simulink model "qdr_ct_test"  (R2012b)
settings: Solver=ode45  StartTime=0.0  StopTime=50000  RelTol=1e-3
libraries: xbsIndex_r4 x1070, casper_library_misc x5, xps_library x4, casper_library_delays x4
(part 1 of 10)
settings Model: Creator=jackh  LastModifiedBy=jackh

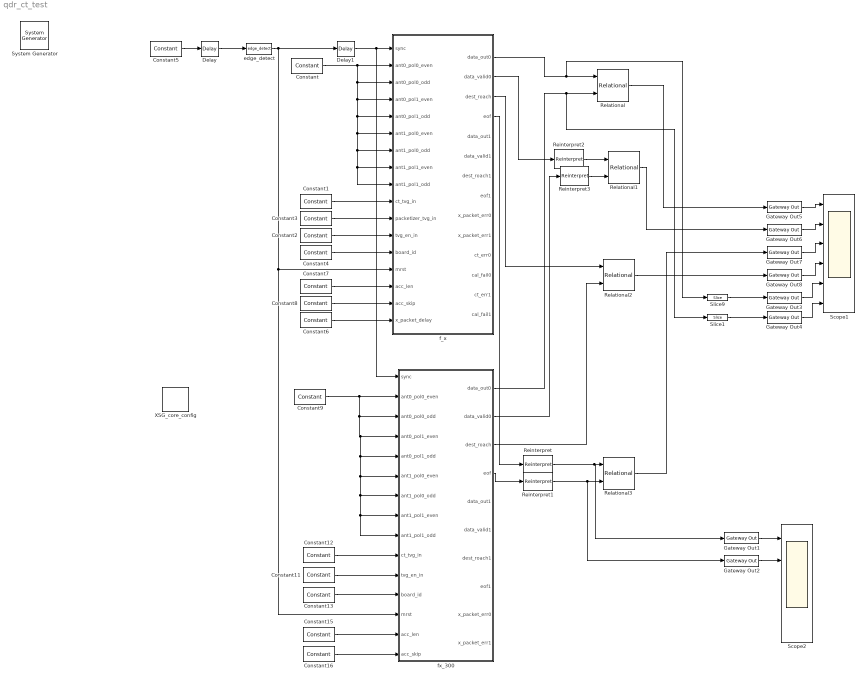
== system qdr_ct_test ==
  " System Generator" : xbsIndex_r4/ System Generator  Tag=genX  xilinxfamily=Kintex7  part=xc7k325t  speed=-3  package=fbg676  synthesis_tool=XST  clock_wrapper=Clock Enables  directory=./netlist  proj_type=Project Navigator  Synth_file=XST Defaults  Impl_file=ISE Defaults  testbench=off  simulink_period=1  sysclk_period=10  dcm_input_clock_period=10  incr_netlist=off  trim_vbits=Everywhere in SubSystem  dbl_ovrd=According to Block Masks  core_generation=According to Block Masks  run_coregen=off  deprecated_control=off  eval_field=0  block_type=sysgen
  Constant{,4,6,9,13} (5 alike) : xbsIndex_r4/Constant  const=0  gui_display_data_type=Fixed-point  arith_type=Unsigned  n_bits=8  bin_pt=0  preci_type=Single  exp_width=8  frac_width=24  explicit_period=on  period=1  equ=P=C  opselect=C  inp2=PCIN>>17  opr=+  inp1=P  carry=CIN  dbl_ovrd=off  block_type=constant
  Constant{1..3,5,11..12} (6 alike) : xbsIndex_r4/Constant  const=1  gui_display_data_type=Boolean  arith_type=Boolean  n_bits=8  bin_pt=0  preci_type=Single  exp_width=8  frac_width=24  explicit_period=on  period=1  equ=P=C  opselect=C  inp2=PCIN>>17  opr=+  inp1=P  carry=CIN  dbl_ovrd=off  block_type=constant
  Constant15 : xbsIndex_r4/Constant  const=64  gui_display_data_type=Fixed-point  arith_type=Unsigned  n_bits=16  bin_pt=0  preci_type=Single  exp_width=8  frac_width=24  explicit_period=on  period=1  equ=P=C  opselect=C  inp2=PCIN>>17  opr=+  inp1=P  carry=CIN  dbl_ovrd=off  block_type=constant
  Constant16 : xbsIndex_r4/Constant  const=10  gui_display_data_type=Fixed-point  arith_type=Unsigned  n_bits=16  bin_pt=0  preci_type=Single  exp_width=8  frac_width=24  explicit_period=on  period=1  equ=P=C  opselect=C  inp2=PCIN>>17  opr=+  inp1=P  carry=CIN  dbl_ovrd=off  block_type=constant
  Constant7 : xbsIndex_r4/Constant  const=32*2  gui_display_data_type=Fixed-point  arith_type=Unsigned  n_bits=16  bin_pt=0  preci_type=Single  exp_width=8  frac_width=24  explicit_period=on  period=1  equ=P=C  opselect=C  inp2=PCIN>>17  opr=+  inp1=P  carry=CIN  dbl_ovrd=off  block_type=constant
  Constant8 : xbsIndex_r4/Constant  const=10  gui_display_data_type=Fixed-point  arith_type=Unsigned  n_bits=16  bin_pt=0  preci_type=Single  exp_width=8  frac_width=24  explicit_period=on  period=1  equ=P=C  opselect=C  inp2=PCIN>>17  opr=+  inp1=P  carry=CIN  dbl_ovrd=off  block_type=constant
  Delay : xbsIndex_r4/Delay  rst=off  infoeditControl=Selection of Reset will increase slice count due to use of real FFs and instead of SRLs  en=off  latency=10  dbl_ovrd=off  reg_retiming=off  block_type=delay
  Delay1 : xbsIndex_r4/Delay  rst=off  infoeditControl=Selection of Reset will increase slice count due to use of real FFs and instead of SRLs  en=off  latency=10  dbl_ovrd=off  reg_retiming=off  block_type=delay
  Gateway Out{1..8} (8 alike) : xbsIndex_r4/Gateway Out  inherit_from_input=off  hdl_port=on  timing_constraint=None  locs_specified=off  LOCs={}  UseAsDAC=off  DACChannel='1'  block_type=gatewayout
  Reinterpret{,1..3} (4 alike) : xbsIndex_r4/Reinterpret  force_arith_type=on  arith_type=Unsigned  force_bin_pt=on  bin_pt=0  block_type=reinterpret
  Relational{,1..3} (4 alike) : xbsIndex_r4/Relational  mode=a=b  en=off  latency=0  dbl_ovrd=off  block_type=relational
  Scope1 : Scope  NumInputPorts=6
      settings: YMin=1~1~1~1~249~249  YMax=1~1~1~1~249~249  SaveName=ScopeData9
  Scope2 : Scope  NumInputPorts=5
      settings: YMin=-5~-5~-5~-5~-5  YMax=5~5~5~5~5  SaveName=ScopeData10
  Slice1 : xbsIndex_r4/Slice  nbits=16  boolean_output=off  mode=Lower Bit Location + Width  bit1=0  base1=MSB of Input  bit0=0  base0=LSB of Input  dbl_ovrd=off  block_type=slice
  Slice9 : xbsIndex_r4/Slice  nbits=16  boolean_output=off  mode=Lower Bit Location + Width  bit1=0  base1=MSB of Input  bit0=0  base0=LSB of Input  dbl_ovrd=off  block_type=slice
  XSG_core_config : xps_library/XSG_core_config  Tag=xps:xsg  hw_sys=ROACH2:sx475t  clk_src=sys_clk  ROACH_clk_src=sys_clk  ROACH2_clk_src=sys_clk  MKDIG_clk_src=sys_clk  clk_rate=100  sample_period=1  synthesis_tool=XST
  edge_detect : casper_library_misc/edge_detect  edge=Rising  polarity=Active High  x_in=[0 0.08 0.08 0.16 0.16 0.24 0.24 0.32 0.32 0.4]  y_in="[-1 -1  1  1  1  1  1  1  1  1]"  x_out=[0.6 0.68 0.68 0.76 0.76 0.84 0.84 0.92 0.92 1]  y_out="[-1 -1  1  1 -1 -1 -1 -1 -1 -1]"
  f_x : Subsystem  mask{fpga_clk=1, fft_size=8, n_pps=50}
      mask prompts: fpga_clk "FPGA Clock (MHz)"; fft_size "FFT channels (2^?)"; n_pps "Accumulations per second"
  fx_300 : Subsystem  mask{fpga_clk=1, fft_size=8, n_pps=50}
      mask prompts: fpga_clk "FPGA Clock (MHz)"; fft_size "FFT channels (2^?)"; n_pps "Accumulations per second"
  wires:
  Constant/1 -> f_x/5(ant0_pol1_odd), f_x/9(ant1_pol1_odd), f_x/8(ant1_pol1_even), f_x/7(ant1_pol0_odd), f_x/6(ant1_pol0_even), f_x/4(ant0_pol1_even), f_x/3(ant0_pol0_odd), f_x/2(ant0_pol0_even)
  Constant1/1 -> f_x/10(ct_tvg_in)
  Constant3/1 -> f_x/11(packetizer_tvg_in)
  Constant2/1 -> f_x/12(tvg_en_in)
  Constant4/1 -> f_x/13(board_id)
  Constant5/1 -> Delay/1
  Delay/1 -> edge_detect/1
  Delay1/1 -> fx_300/1(sync), f_x/1(sync)
  Constant6/1 -> f_x/17(x_packet_delay)
  Constant7/1 -> f_x/15(acc_len)
  Constant8/1 -> f_x/16(acc_skip)
  Constant9/1 -> fx_300/9(ant1_pol1_odd), fx_300/8(ant1_pol1_even), fx_300/7(ant1_pol0_odd), fx_300/6(ant1_pol0_even), fx_300/5(ant0_pol1_odd), fx_300/4(ant0_pol1_even), fx_300/3(ant0_pol0_odd), fx_300/2(ant0_pol0_even)
  Constant12/1 -> fx_300/10(ct_tvg_in)
  Constant11/1 -> fx_300/11(tvg_en_in)
  Constant13/1 -> fx_300/12(board_id)
  edge_detect/1 -> fx_300/13(mrst), f_x/14(mrst), Delay1/1
  Constant15/1 -> fx_300/14(acc_len)
  Constant16/1 -> fx_300/15(acc_skip)
  fx_300/1(data_out0) -> Slice1/1, Relational/2
  f_x/1(data_out0) -> Slice9/1, Relational/1
  f_x/2(data_valid0) -> Reinterpret2/1
  fx_300/2(data_valid0) -> Reinterpret3/1
  f_x/3(dest_roach) -> Relational2/1
  fx_300/3(dest_roach) -> Relational2/2
  f_x/4(eof) -> Reinterpret/1
  fx_300/4(eof) -> Reinterpret1/1
  Gateway Out6/1 -> Scope1/2
  Gateway Out3/1 -> Scope1/5
  Gateway Out7/1 -> Scope1/3
  Gateway Out5/1 -> Scope1/1
  Gateway Out8/1 -> Scope1/4
  Relational/1 -> Gateway Out5/1
  Relational1/1 -> Gateway Out6/1
  Relational2/1 -> Gateway Out7/1
  Relational3/1 -> Gateway Out8/1
  Gateway Out2/1 -> Scope2/2
  ? -> Scope2/5
  ? -> Scope2/3
  Gateway Out1/1 -> Scope2/1
  ? -> Scope2/4
  Reinterpret/1 -> Gateway Out1/1, Relational3/1
  Reinterpret1/1 -> Gateway Out2/1, Relational3/2
  Reinterpret2/1 -> Relational1/1
  Reinterpret3/1 -> Relational1/2
  Gateway Out4/1 -> Scope1/6
  Slice9/1 -> Gateway Out3/1
  Slice1/1 -> Gateway Out4/1
